simulink model "adarbha_HW8_sim"  (Simulink 7.7)
settings: Solver=ode4  StartTime=0.0  StopTime=max(Time)  RelTol=1e-3
values from neighbouring files (symbols this model uses):
  Area_sq_m = 2.4    [adarbha_HW8.m]
  Cd = 0.40    (= 0.4)    [Coast_Down_Initial_AJ.m]    (also in adarbha_HW8.m = (2*Mass_kg*beta(j)*atan(beta(j))/(rho*Area_sq_m*Velocity_mps)
  rho = 1.24    [Coast_Down_Initial_AJ.m]    (also in adarbha_HW8.m)
  Time = [Time T_final]    [adarbha_HW8.m]
  Vel_sim = vel_ratio_sim*Velocity_mps(1)    [adarbha_HW8.m]
  Velocity_mps = [Velocity_mps 0]    [adarbha_HW8.m]
  Weight_N = 18680    [Coast_Down_Initial_AJ.m]    (also in adarbha_HW8.m)
  wheel_radius = 0.318    [adarbha_HW8.m]
settings Model: Creator=Arjun  LastModifiedBy=Arjun

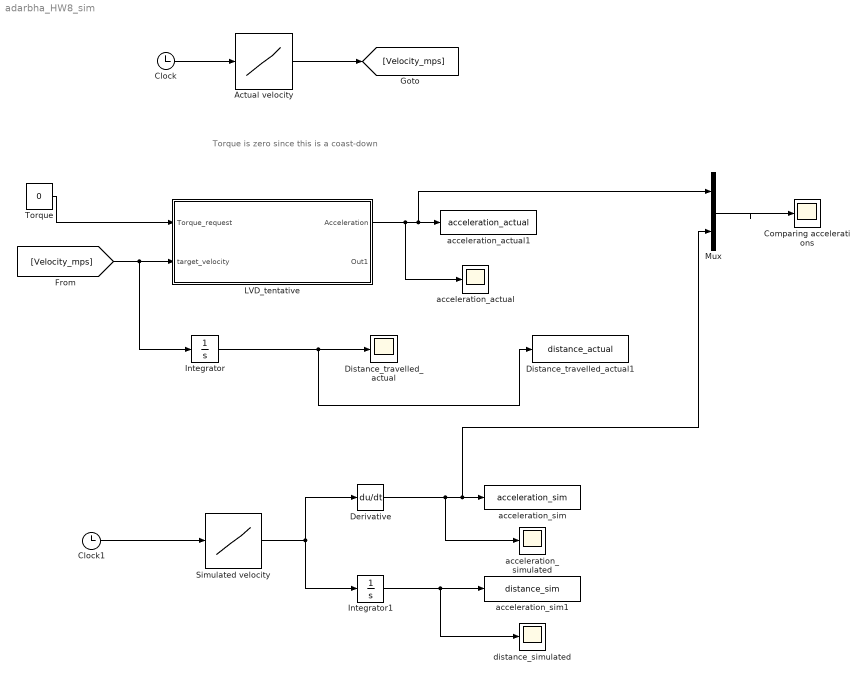
== system adarbha_HW8_sim ==
  note: Torque is zero since this is a coast-down
  Actual velocity : Lookup_n-D  NumberOfTableDimensions=1  BreakpointsForDimension1=Time  Table=Velocity_mps  RndMeth=Simplest  InputSameDT=on
  Clock : Clock
      settings: Decimation=10
  Clock1 : Clock
      settings: Decimation=10
  Comparing accelerations : Scope
      settings: SaveName=ScopeData4
  Derivative : Derivative
  Distance_travelled_actual : Scope
  Distance_travelled_actual1 : ToWorkspace  VariableName=distance_actual  SampleTime=-1  SaveFormat=Structure
  Integrator : Integrator
  Integrator1 : Integrator
  LVD_tentative : Subsystem
  Mux : Mux  Inputs=2
  Simulated velocity : Lookup_n-D  NumberOfTableDimensions=1  BreakpointsForDimension1=Time  Table=Vel_sim  RndMeth=Simplest  InputSameDT=on
  Torque : Constant  Value=0
  acceleration_actual : Scope
  acceleration_actual1 : ToWorkspace  VariableName=acceleration_actual  SampleTime=-1  SaveFormat=Structure
  acceleration_sim : ToWorkspace  VariableName=acceleration_sim  SampleTime=-1  SaveFormat=Structure
  acceleration_sim1 : ToWorkspace  VariableName=distance_sim  SampleTime=-1  SaveFormat=Structure
  acceleration_simulated : Scope
      settings: SaveName=ScopeData2
  distance_simulated : Scope
      settings: SaveName=ScopeData3
  wires:
  Clock/1 -> Actual velocity/1
  Integrator/1 -> Distance_travelled_actual/1, Distance_travelled_actual1/1
  Torque/1 -> LVD_tentative/1(Torque_request)
  Actual velocity/1 -> [Velocity_mps]
  [Velocity_mps] -> LVD_tentative/2(target_velocity), Integrator/1
  LVD_tentative/1(Acceleration) -> acceleration_actual/1, acceleration_actual1/1, Mux/1
  Clock1/1 -> Simulated velocity/1
  Simulated velocity/1 -> Derivative/1, Integrator1/1
  Derivative/1 -> acceleration_simulated/1, acceleration_sim/1, Mux/2
  Integrator1/1 -> acceleration_sim1/1, distance_simulated/1
  Mux/1 -> Comparing accelerations/1

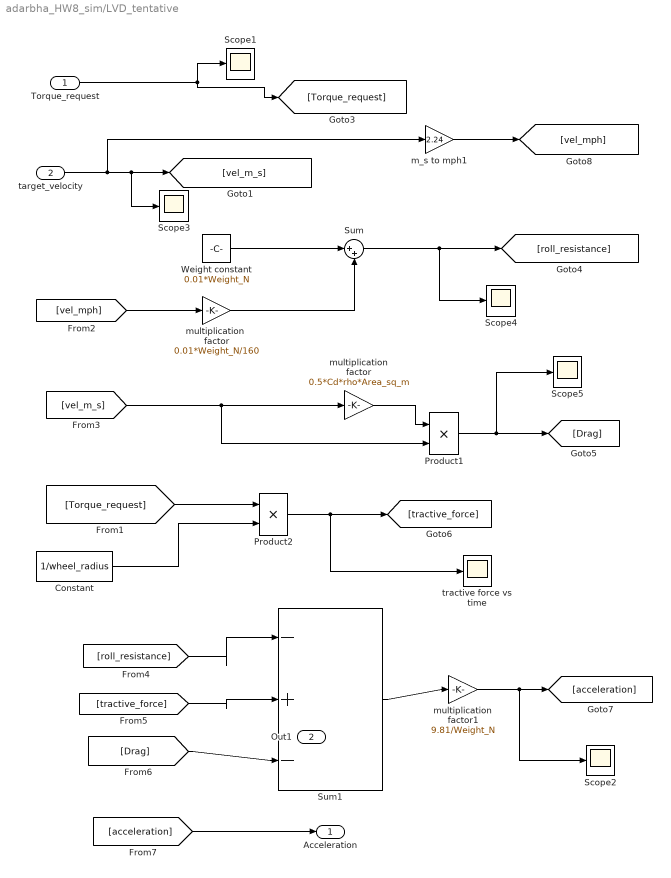
== system adarbha_HW8_sim/LVD_tentative ==
  Torque_request : Inport
  target_velocity : Inport  Port=2
  Constant : Constant  Value=1/wheel_radius
  Product1 : Product  RndMeth=Zero
  Product2 : Product  RndMeth=Zero
  Scope{1..5} (5 alike) : Scope
      Scope1 settings: SaveName=ScopeData5
      Scope2 settings: SaveName=ScopeData6
      Scope3 settings: SaveName=ScopeData8
      Scope4 settings: SaveName=ScopeData9
      Scope5 settings: SaveName=ScopeData10
  Sum : Sum  Inputs=|++
  Sum1 : Sum  Inputs=|-+-
  Weight constant : Constant  Value=0.01*Weight_N
  m_s to mph1 : Gain  Gain=2.24
  multiplication  factor : Gain  Gain=0.01*Weight_N/160
  multiplication factor : Gain  Gain=0.5*Cd*rho*Area_sq_m
  multiplication factor1 : Gain  Gain=9.81/Weight_N
  tractive force vs time : Scope
      settings: SaveName=ScopeData13
  Acceleration : Outport
  Out1 : Outport  Port=2
  wires:
  Weight constant/1 -> Sum/1
  multiplication  factor/1 -> Sum/2
  Sum/1 -> [roll_resistance], Scope4/1
  [vel_mph] -> multiplication  factor/1
  multiplication factor/1 -> Product1/1
  [vel_m_s] -> multiplication factor/1, Product1/2
  Product1/1 -> [Drag], Scope5/1
  [Torque_request] -> Product2/1
  Constant/1 -> Product2/2
  Product2/1 -> [tractive_force], tractive force vs time/1
  [roll_resistance] -> Sum1/1
  [tractive_force] -> Sum1/2
  [Drag] -> Sum1/3
  Sum1/1 -> multiplication factor1/1
  multiplication factor1/1 -> [acceleration], Scope2/1
  Torque_request/1 -> [Torque_request], Scope1/1
  target_velocity/1 -> m_s to mph1/1, [vel_m_s], Scope3/1
  m_s to mph1/1 -> [vel_mph]
  [acceleration] -> Acceleration/1
